simulink model "CPM_f0_v2"  (R2023a)
settings: Solver=VariableStepAuto  StartTime=0.0  StopTime=6  RelTol=1e-3
values from neighbouring files (symbols this model uses):
  A = sqrt(2*E/sampleTime)    [dataCPM.m]
  f_0 = 2*pi*200    (= 1256.63706144)    [dataCPM.m]
  f_1 = f_0 + f    (= 1258.20785776)    [dataCPM.m]
  f_2 = f_0 - f    (= 1255.06626511)    [dataCPM.m]
  sample_n = 500    [dataCPM.m]
  sampleTime = 1    [dataCPM.m]
undefined symbols (not defined in the file or in its folder): DiscIntNeverNeededParam
libraries: simulink x9, simulink_extras x4, commdigbbndcpm2 x2
settings Model: Creator=mluser  LastModifiedBy=x
settings DebuggingCC: ParameterOverflowMsg=none  ParameterUnderflowMsg=error

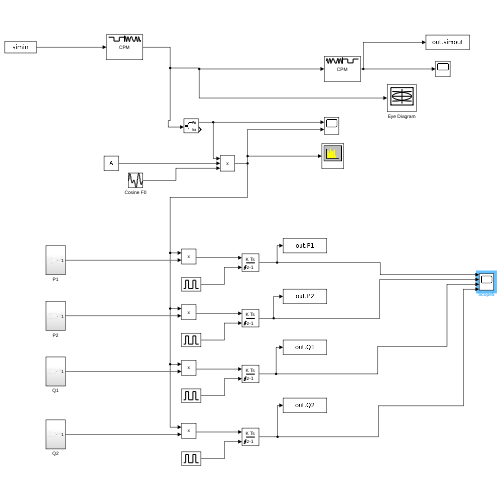
[thumbnail: Simulink's stored preview of the top-level diagram]
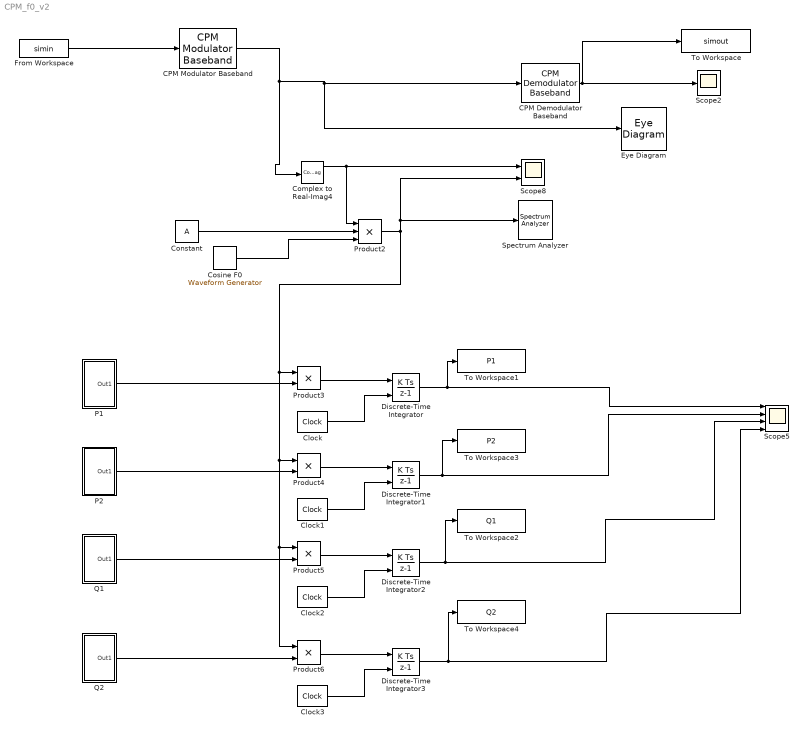
== system CPM_f0_v2 ==
  CPM Demodulator Baseband : commdigbbndcpm2/CPM Demodulator Baseband  Mnum=2  outputType=Integer  mappingType=Binary  modIdx=0.5  pulseShape=Rectangular  BT=0.3  mainLobePulseLength=1  rollOff=0.2  pulseLength=1  preHistory=1  phaseOffset=0  samplesPerSymbol=sample_n  RateOptions=Allow multirate processing  traceBack=1  outDType=double
  CPM Modulator Baseband : commdigbbndcpm2/CPM Modulator Baseband  Mnum=2  inputType=Integer  mappingType=Binary  modIdx=0.5  pulseShape=Rectangular  BT=0.3  mainLobePulseLength=1  rollOff=0.2  pulseLength=1  preHistory=1  phaseOffset=0  samplesPerSymbol=sample_n  RateOptions=Allow multirate processing  outDataType=double
  Clock{,1..3} (4 alike) : simulink_extras/Flip Flops/Clock  period=sampleTime+0.000001
  Complex to Real-Imag4 : ComplexToRealImag
  Constant : Constant  Value=A
  Cosine F0 : simulink/Sources/Waveform Generator  OutMin=[]  OutMax=[]  OutDataTypeStr=double  SelectedSignal=1  Signals=sin(A, f_0, pi/2)  BlockNames=MultiportSwitch_26b22544997148d  SampleTime=1/sample_n
  Discrete-Time Integrator{,1..3} (4 alike) : DiscreteIntegrator  ExternalReset=rising  SampleTime=1/sample_n  OutDataTypeStr=double  ICPrevOutput=DiscIntNeverNeededParam  ICPrevScaledInput=DiscIntNeverNeededParam
  Eye Diagram : EyeDiagram
  From Workspace : FromWorkspace  VariableName=simin  OutDataTypeStr=double  SampleTime=sampleTime  Interpolate=off  OutputAfterFinalValue=Holding final value
  P1 : Subsystem
  P2 : Subsystem
  Product2 : Product  Inputs=3
  Product{3..6} (4 alike) : Product
  Q1 : Subsystem
  Q2 : Subsystem
  Scope2 : Scope
  Scope5 : Scope  NumInputPorts=4
  Scope8 : Scope  NumInputPorts=2
  Spectrum Analyzer : SpectrumAnalyzer  WindowPosition=[560.000000,290.000000,800.000000,500.000000,]  ScopeFrameLocation=window  Span=5000  StartFrequency=-2500  StopFrequency=2500  YLimits=[-180.25709895,-62.31219254]  ColorLimits=[-80 20]
  To Workspace : ToWorkspace  VariableName=simout  SampleTime=-1
      settings: Save2DSignal=2-D array (concatenate along first dimension)
  To Workspace1 : ToWorkspace  VariableName=P1  SampleTime=1
      settings: Save2DSignal=2-D array (concatenate along first dimension)
  To Workspace2 : ToWorkspace  VariableName=Q1  SampleTime=1
      settings: Save2DSignal=2-D array (concatenate along first dimension)
  To Workspace3 : ToWorkspace  VariableName=P2  SampleTime=1
      settings: Save2DSignal=2-D array (concatenate along first dimension)
  To Workspace4 : ToWorkspace  VariableName=Q2  SampleTime=1
      settings: Save2DSignal=2-D array (concatenate along first dimension)
  wires:
  From Workspace/1 -> CPM Modulator Baseband/1
  CPM Demodulator Baseband/1 -> To Workspace/1, Scope2/1
  CPM Modulator Baseband/1 -> Complex to Real-Imag4/1, Eye Diagram/1, CPM Demodulator Baseband/1
  Constant/1 -> Product2/2
  Product2/1 -> Product6/1, Product5/1, Product4/1, Product3/1, Scope8/2, Spectrum Analyzer/1
  Q2/1(Out1) -> Product6/2
  Q1/1(Out1) -> Product5/2
  P2/1(Out1) -> Product4/2
  P1/1(Out1) -> Product3/2
  Discrete-Time Integrator/1 -> To Workspace1/1, Scope5/1
  Discrete-Time Integrator1/1 -> To Workspace3/1, Scope5/2
  Discrete-Time Integrator2/1 -> To Workspace2/1, Scope5/3
  Discrete-Time Integrator3/1 -> To Workspace4/1, Scope5/4
  Cosine F0/1 -> Product2/3
  Product3/1 -> Discrete-Time Integrator/1
  Complex to Real-Imag4/1 -> Product2/1, Scope8/1
  Clock/1 -> Discrete-Time Integrator/2
  Product4/1 -> Discrete-Time Integrator1/1
  Clock1/1 -> Discrete-Time Integrator1/2
  Product5/1 -> Discrete-Time Integrator2/1
  Clock2/1 -> Discrete-Time Integrator2/2
  Product6/1 -> Discrete-Time Integrator3/1
  Clock3/1 -> Discrete-Time Integrator3/2

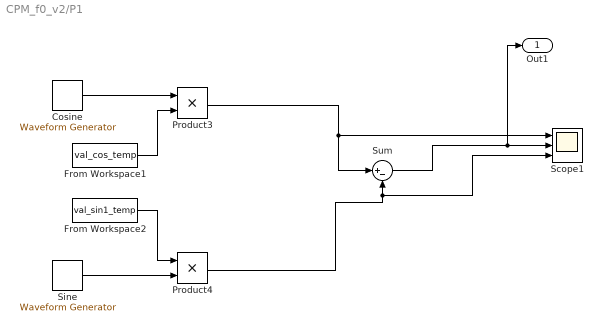
== system CPM_f0_v2/P1 ==
  Cosine : simulink/Sources/Waveform Generator  OutMin=[]  OutMax=[]  OutDataTypeStr=double  SelectedSignal=1  Signals=sin(A,f_1,pi/2)  BlockNames=MultiportSwitch_25698e59d6fd41e  SampleTime=1/sample_n
  From Workspace1 : FromWorkspace  VariableName=val_cos_temp  SampleTime=sampleTime  OutputAfterFinalValue=Holding final value
  From Workspace2 : FromWorkspace  VariableName=val_sin1_temp  SampleTime=sampleTime  OutputAfterFinalValue=Holding final value
  Product3 : Product
  Product4 : Product
  Scope1 : Scope  NumInputPorts=3
  Sine : simulink/Sources/Waveform Generator  OutMin=[]  OutMax=[]  OutDataTypeStr=double  SelectedSignal=1  Signals=sin(A,f_1,0)  BlockNames=MultiportSwitch_18ea0db491b64bb  SampleTime=1/sample_n
  Sum : Sum  Inputs=|+-
  Out1 : Outport
  wires:
  Sum/1 -> Out1/1, Scope1/2
  From Workspace1/1 -> Product3/2
  Product4/1 -> Scope1/3, Sum/2
  Product3/1 -> Sum/1, Scope1/1
  From Workspace2/1 -> Product4/1
  Sine/1 -> Product4/2
  Cosine/1 -> Product3/1

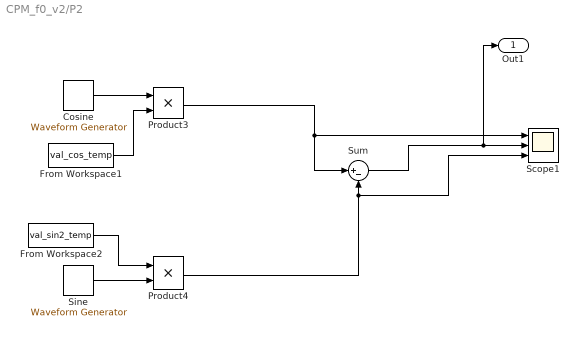
== system CPM_f0_v2/P2 ==
  Cosine : simulink/Sources/Waveform Generator  OutMin=[]  OutMax=[]  OutDataTypeStr=double  SelectedSignal=1  Signals=sin(A,f_2,pi/2)  BlockNames=MultiportSwitch_8e5bdfc73f064c2  SampleTime=1/sample_n
  From Workspace1 : FromWorkspace  VariableName=val_cos_temp  SampleTime=sampleTime  OutputAfterFinalValue=Holding final value
  From Workspace2 : FromWorkspace  VariableName=val_sin2_temp  SampleTime=sampleTime  OutputAfterFinalValue=Holding final value
  Product3 : Product
  Product4 : Product
  Scope1 : Scope  NumInputPorts=3
  Sine : simulink/Sources/Waveform Generator  OutMin=[]  OutMax=[]  OutDataTypeStr=double  SelectedSignal=1  Signals=sin(A,f_2,0)  BlockNames=MultiportSwitch_322871e150d44c1  SampleTime=1/sample_n
  Sum : Sum  Inputs=|+-
  Out1 : Outport
  wires:
  Sum/1 -> Out1/1, Scope1/2
  From Workspace1/1 -> Product3/2
  Cosine/1 -> Product3/1
  Sine/1 -> Product4/2
  Product4/1 -> Scope1/3, Sum/2
  Product3/1 -> Sum/1, Scope1/1
  From Workspace2/1 -> Product4/1

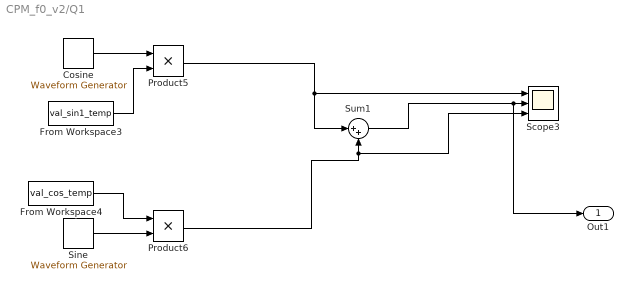
== system CPM_f0_v2/Q1 ==
  Cosine : simulink/Sources/Waveform Generator  OutMin=[]  OutMax=[]  OutDataTypeStr=double  SelectedSignal=1  Signals=sin(A,f_1,pi/2)  BlockNames=MultiportSwitch_25698e59d6fd41e  SampleTime=1/sample_n
  From Workspace3 : FromWorkspace  VariableName=val_sin1_temp  SampleTime=sampleTime  OutputAfterFinalValue=Holding final value
  From Workspace4 : FromWorkspace  VariableName=val_cos_temp  SampleTime=sampleTime  OutputAfterFinalValue=Holding final value
  Product5 : Product
  Product6 : Product
  Scope3 : Scope  NumInputPorts=3
  Sine : simulink/Sources/Waveform Generator  OutMin=[]  OutMax=[]  OutDataTypeStr=double  SelectedSignal=1  Signals=sin(A,f_1,0)  BlockNames=MultiportSwitch_18ea0db491b64bb  SampleTime=1/sample_n
  Sum1 : Sum  Inputs=|++
  Out1 : Outport
  wires:
  From Workspace3/1 -> Product5/2
  Sine/1 -> Product6/2
  Cosine/1 -> Product5/1
  From Workspace4/1 -> Product6/1
  Product6/1 -> Scope3/3, Sum1/2
  Sum1/1 -> Out1/1, Scope3/2
  Product5/1 -> Sum1/1, Scope3/1

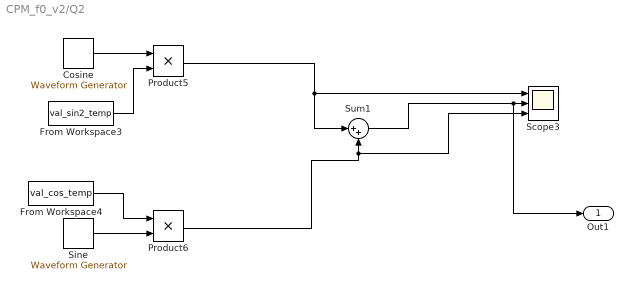
== system CPM_f0_v2/Q2 ==
  Cosine : simulink/Sources/Waveform Generator  OutMin=[]  OutMax=[]  OutDataTypeStr=double  SelectedSignal=1  Signals=sin(A,f_2,pi/2)  BlockNames=MultiportSwitch_6109da47d17e4ad  SampleTime=1/sample_n
  From Workspace3 : FromWorkspace  VariableName=val_sin2_temp  SampleTime=sampleTime  OutputAfterFinalValue=Holding final value
  From Workspace4 : FromWorkspace  VariableName=val_cos_temp  SampleTime=sampleTime  OutputAfterFinalValue=Holding final value
  Product5 : Product
  Product6 : Product
  Scope3 : Scope  NumInputPorts=3
  Sine : simulink/Sources/Waveform Generator  OutMin=[]  OutMax=[]  OutDataTypeStr=double  SelectedSignal=1  Signals=sin(A,f_2,0)  BlockNames=MultiportSwitch_bb487db733a9414  SampleTime=1/sample_n
  Sum1 : Sum  Inputs=|++
  Out1 : Outport
  wires:
  From Workspace3/1 -> Product5/2
  Sine/1 -> Product6/2
  Cosine/1 -> Product5/1
  From Workspace4/1 -> Product6/1
  Product6/1 -> Scope3/3, Sum1/2
  Sum1/1 -> Out1/1, Scope3/2
  Product5/1 -> Sum1/1, Scope3/1
